simulink model "gm_sampleModel66206_pp_7_1_sub"  (R2023b)
settings: Solver=VariableStepAuto  StartTime=0.0  StopTime=10.0  RelTol=1e-3
libraries: simulink x38, hdlsllib x2, hdlmdlgenlib x2
(part 2 of 2)

== system gm_sampleModel66206_pp_7_1_sub/Subsystem/cfblk35 ==
  emi_178 : Inport  OutDataTypeStr=uint8  PortDimensions=1  SampleTime=1
  Action Port : Inport  Port=2  OutDataTypeStr=boolean  SampleTime=1
  Reshape : Reshape
  cfblk35_out1bypassMux : MultiPortSwitch  DataPortOrder=Zero-based contiguous  Inputs=2  zeroidx=on  OutDataTypeStr=uint8  SampleTime=1  SaturateOnIntegerOverflow=off  InputSameDT=off
  emi_179_bypass : UnitDelay  InitialCondition="fi(0,0,8,0,\"hex\",\"00\")"  SampleTime=1
  emi_179 : Outport  SampleTime=1  InitialOutput=0
  wires:
  Action Port/1 -> cfblk35_out1bypassMux/1
  emi_178/1 -> Reshape/1
  Reshape/1 -> cfblk35_out1bypassMux/3
  cfblk35_out1bypassMux/1 -> emi_179_bypass/1, emi_179/1
  emi_179_bypass/1 -> cfblk35_out1bypassMux/2

== system gm_sampleModel66206_pp_7_1_sub/Subsystem/cfblk36_inst ==
  in1 : Inport  OutDataTypeStr=uint8  SampleTime=1
  in2 : Inport  Port=2  OutDataTypeStr=uint8  SampleTime=1
  mul_cfblk36_dotp_mulcomp : Product  Inputs=**  OutDataTypeStr=uint8  SampleTime=1
  out1 : Outport  OutDataTypeStr=uint8  SampleTime=1
  wires:
  in1/1 -> mul_cfblk36_dotp_mulcomp/1
  in2/1 -> mul_cfblk36_dotp_mulcomp/2
  mul_cfblk36_dotp_mulcomp/1 -> out1/1

== system gm_sampleModel66206_pp_7_1_sub/Subsystem/cfblk40 ==
  u : Inport  OutDataTypeStr=uint8  SampleTime=1
  FixPt Constant : Constant  DisableCoverage=on  OutDataTypeStr=Inherit: Inherit via back propagation  SampleTime=-1
  FixPt Data Type Duplicate : DataTypeDuplicate  DisableCoverage=on  NumInputPorts=3
  FixPt Sum1 : Sum  OutDataTypeStr=Inherit: Inherit via back propagation  InputSameDT=on  LockScale=on
  y : Outport  SampleTime=1
  wires:
  u/1 -> FixPt Sum1/1, FixPt Data Type Duplicate/2
  FixPt Constant/1 -> FixPt Sum1/2, FixPt Data Type Duplicate/3
  FixPt Sum1/1 -> FixPt Data Type Duplicate/1, y/1

== system gm_sampleModel66206_pp_7_1_sub/Subsystem/cfblk42_inst ==
  in1 : Inport  OutDataTypeStr=uint8  SampleTime=1
  in2 : Inport  Port=2  OutDataTypeStr=uint8  SampleTime=1
  mul_cfblk42_dotp_mulcomp : Product  Inputs=**  OutDataTypeStr=uint8  SampleTime=1
  out1 : Outport  OutDataTypeStr=uint8  SampleTime=1
  wires:
  in1/1 -> mul_cfblk42_dotp_mulcomp/1
  in2/1 -> mul_cfblk42_dotp_mulcomp/2
  mul_cfblk42_dotp_mulcomp/1 -> out1/1

== system gm_sampleModel66206_pp_7_1_sub/Subsystem/cfblk44_inst ==
  in1 : Inport  OutDataTypeStr=uint8  SampleTime=1
  in2 : Inport  Port=2  OutDataTypeStr=uint8  SampleTime=1
  mul_cfblk44_dotp_mulcomp : Product  Inputs=**  OutDataTypeStr=uint8  SampleTime=1
  out1 : Outport  OutDataTypeStr=uint8  SampleTime=1
  wires:
  in1/1 -> mul_cfblk44_dotp_mulcomp/1
  in2/1 -> mul_cfblk44_dotp_mulcomp/2
  mul_cfblk44_dotp_mulcomp/1 -> out1/1

== system gm_sampleModel66206_pp_7_1_sub/Subsystem/cfblk47 ==
  emi_186 : Inport  OutDataTypeStr=uint8  PortDimensions=1  SampleTime=1
  Action Port : Inport  Port=2  OutDataTypeStr=boolean  SampleTime=1
  cfblk47 : Sum  Inputs=+
  cfblk47_out1bypassMux : MultiPortSwitch  DataPortOrder=Zero-based contiguous  Inputs=2  zeroidx=on  OutDataTypeStr=uint8  SampleTime=1  SaturateOnIntegerOverflow=off  InputSameDT=off
  emi_187_bypass : UnitDelay  InitialCondition="fi(0,0,8,0,\"hex\",\"00\")"  SampleTime=1
  emi_187 : Outport  SampleTime=1  InitialOutput=0
  wires:
  Action Port/1 -> cfblk47_out1bypassMux/1
  emi_186/1 -> cfblk47/1
  cfblk47/1 -> cfblk47_out1bypassMux/3
  cfblk47_out1bypassMux/1 -> emi_187_bypass/1, emi_187/1
  emi_187_bypass/1 -> cfblk47_out1bypassMux/2

== system gm_sampleModel66206_pp_7_1_sub/Subsystem/cfblk5 ==
  emi_202 : Inport  OutDataTypeStr=fixdt(0, 16, 7)  PortDimensions=1  SampleTime=1
  Action Port : Inport  Port=2  OutDataTypeStr=boolean  SampleTime=1
  cfblk5 : Subsystem  mask(Detect Fall Nonpositive){vinit=double(0), InputProcessing=Elements as channels (sample based), OutDataTypeStr=uint8}
      mask prompts: vinit "Simulink:masks:InitialCondition_MP"; InputProcessing "Simulink:masks:InputProcessing_MP"; OutDataTypeStr "Simulink:masks:OutputDataType_MP"
      mask help: Simulink:masks:DetectFallNonpositive_MD
      mask TypeOptions InputProcessing: Simulink:masks:ColumnsAsChannelsFrameBased | Simulink:masks:ElementsAsChannelsSampleBased
      mask TypeOptions OutDataTypeStr: Simulink:masks:uint8 | Simulink:masks:boolean
      mask Display: fprintf('U <= 0\n&  NOT\nU/z <= 0')
  cfblk5_out1bypassMux : MultiPortSwitch  DataPortOrder=Zero-based contiguous  Inputs=2  zeroidx=on  OutDataTypeStr=uint8  SampleTime=1  SaturateOnIntegerOverflow=off  InputSameDT=off
  emi_203_bypass : UnitDelay  InitialCondition="fi(0,0,8,0,\"hex\",\"00\")"  SampleTime=1
  emi_203 : Outport  SampleTime=1  InitialOutput=0
  wires:
  Action Port/1 -> cfblk5_out1bypassMux/1, cfblk5/2(Action Port_out2)
  emi_202/1 -> cfblk5/1(U)
  cfblk5/1(Y) -> cfblk5_out1bypassMux/3
  cfblk5_out1bypassMux/1 -> emi_203_bypass/1, emi_203/1
  emi_203_bypass/1 -> cfblk5_out1bypassMux/2

== system gm_sampleModel66206_pp_7_1_sub/Subsystem/cfblk50 ==
  emi_210 : Inport  OutDataTypeStr=uint8  PortDimensions=1  SampleTime=1
  Action Port : Inport  Port=2  OutDataTypeStr=boolean  SampleTime=1
  cfblk50 : Gain  Gain="fi(0,0,8,7,\"hex\",\"80\")"  ParamDataTypeStr=fixdt(0, 8, 7)  OutDataTypeStr=fixdt(0, 16, 7)  SampleTime=1
  cfblk50_out1bypassMux : MultiPortSwitch  DataPortOrder=Zero-based contiguous  Inputs=2  zeroidx=on  OutDataTypeStr=fixdt(0, 16, 7)  SampleTime=1  SaturateOnIntegerOverflow=off  InputSameDT=off
  emi_211_bypass : UnitDelay  InitialCondition="fi(0,0,16,7,\"hex\",\"0000\")"  SampleTime=1
  emi_211 : Outport  SampleTime=1  InitialOutput=0
  wires:
  Action Port/1 -> cfblk50_out1bypassMux/1
  emi_210/1 -> cfblk50/1
  cfblk50/1 -> cfblk50_out1bypassMux/3
  cfblk50_out1bypassMux/1 -> emi_211_bypass/1, emi_211/1
  emi_211_bypass/1 -> cfblk50_out1bypassMux/2

== system gm_sampleModel66206_pp_7_1_sub/Subsystem/cfblk51 ==
  emi_218 : Inport  OutDataTypeStr=uint8  PortDimensions=1  SampleTime=1
  Action Port : Inport  Port=2  OutDataTypeStr=boolean  SampleTime=1
  cfblk51 : Subsystem  mask(Real World Value Increment){}
      mask help: Simulink:masks:RealWorldValueIncrement_MD
      mask Display: disp('V++')
  cfblk51_out1bypassMux : MultiPortSwitch  DataPortOrder=Zero-based contiguous  Inputs=2  zeroidx=on  OutDataTypeStr=uint8  SampleTime=1  SaturateOnIntegerOverflow=off  InputSameDT=off
  emi_219_bypass : UnitDelay  InitialCondition="fi(0,0,8,0,\"hex\",\"00\")"  SampleTime=1
  emi_219 : Outport  SampleTime=1  InitialOutput=0
  wires:
  Action Port/1 -> cfblk51_out1bypassMux/1
  emi_218/1 -> cfblk51/1(u)
  cfblk51/1(y) -> cfblk51_out1bypassMux/3
  cfblk51_out1bypassMux/1 -> emi_219_bypass/1, emi_219/1
  emi_219_bypass/1 -> cfblk51_out1bypassMux/2

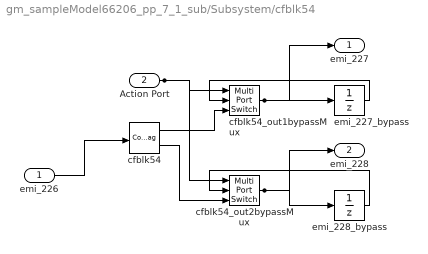
== system gm_sampleModel66206_pp_7_1_sub/Subsystem/cfblk54 ==
  emi_226 : Inport  OutDataTypeStr=uint8  PortDimensions=1  SampleTime=1
  Action Port : Inport  Port=2  OutDataTypeStr=boolean  SampleTime=1
  cfblk54 : ComplexToRealImag  SampleTime=1
  cfblk54_out1bypassMux : MultiPortSwitch  DataPortOrder=Zero-based contiguous  Inputs=2  zeroidx=on  OutDataTypeStr=uint8  SampleTime=1  SaturateOnIntegerOverflow=off  InputSameDT=off
  cfblk54_out2bypassMux : MultiPortSwitch  DataPortOrder=Zero-based contiguous  Inputs=2  zeroidx=on  OutDataTypeStr=uint8  SampleTime=1  SaturateOnIntegerOverflow=off  InputSameDT=off
  emi_227_bypass : UnitDelay  InitialCondition="fi(0,0,8,0,\"hex\",\"00\")"  SampleTime=1
  emi_228_bypass : UnitDelay  InitialCondition="fi(0,0,8,0,\"hex\",\"00\")"  SampleTime=1
  emi_227 : Outport  SampleTime=1  InitialOutput=0
  emi_228 : Outport  Port=2  SampleTime=1  InitialOutput=0
  wires:
  Action Port/1 -> cfblk54_out2bypassMux/1, cfblk54_out1bypassMux/1
  emi_226/1 -> cfblk54/1
  cfblk54/1 -> cfblk54_out1bypassMux/3
  cfblk54/2 -> cfblk54_out2bypassMux/3
  cfblk54_out1bypassMux/1 -> emi_227_bypass/1, emi_227/1
  emi_227_bypass/1 -> cfblk54_out1bypassMux/2
  cfblk54_out2bypassMux/1 -> emi_228_bypass/1, emi_228/1
  emi_228_bypass/1 -> cfblk54_out2bypassMux/2

== system gm_sampleModel66206_pp_7_1_sub/Subsystem/cfblk55 ==
  emi_235 : Inport  OutDataTypeStr=uint8  PortDimensions=1  SampleTime=1
  Action Port : Inport  Port=2  OutDataTypeStr=boolean  SampleTime=1
  cfblk55 : Abs  SampleTime=1  OutDataTypeStr=uint8  SaturateOnIntegerOverflow=off
  cfblk55_out1bypassMux : MultiPortSwitch  DataPortOrder=Zero-based contiguous  Inputs=2  zeroidx=on  OutDataTypeStr=uint8  SampleTime=1  SaturateOnIntegerOverflow=off  InputSameDT=off
  emi_236_bypass : UnitDelay  InitialCondition="fi(0,0,8,0,\"hex\",\"00\")"  SampleTime=1
  emi_236 : Outport  SampleTime=1  InitialOutput=0
  wires:
  Action Port/1 -> cfblk55_out1bypassMux/1
  emi_235/1 -> cfblk55/1
  cfblk55/1 -> cfblk55_out1bypassMux/3
  cfblk55_out1bypassMux/1 -> emi_236_bypass/1, emi_236/1
  emi_236_bypass/1 -> cfblk55_out1bypassMux/2

== system gm_sampleModel66206_pp_7_1_sub/Subsystem/cfblk59 ==
  u : Inport  OutDataTypeStr=uint8  SampleTime=1
  FixPt Constant : Constant  DisableCoverage=on  OutDataTypeStr=Inherit: Inherit via back propagation  SampleTime=-1
  FixPt Data Type Duplicate : DataTypeDuplicate  DisableCoverage=on  NumInputPorts=3
  FixPt Sum1 : Sum  OutDataTypeStr=Inherit: Inherit via back propagation  InputSameDT=on  LockScale=on
  y : Outport  SampleTime=1
  wires:
  u/1 -> FixPt Sum1/1, FixPt Data Type Duplicate/2
  FixPt Constant/1 -> FixPt Sum1/2, FixPt Data Type Duplicate/3
  FixPt Sum1/1 -> FixPt Data Type Duplicate/1, y/1

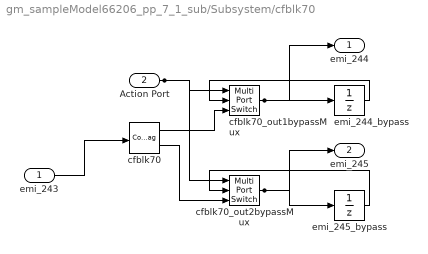
== system gm_sampleModel66206_pp_7_1_sub/Subsystem/cfblk70 ==
  emi_243 : Inport  OutDataTypeStr=uint8  PortDimensions=1  SampleTime=1
  Action Port : Inport  Port=2  OutDataTypeStr=boolean  SampleTime=1
  cfblk70 : ComplexToRealImag  SampleTime=1
  cfblk70_out1bypassMux : MultiPortSwitch  DataPortOrder=Zero-based contiguous  Inputs=2  zeroidx=on  OutDataTypeStr=uint8  SampleTime=1  SaturateOnIntegerOverflow=off  InputSameDT=off
  cfblk70_out2bypassMux : MultiPortSwitch  DataPortOrder=Zero-based contiguous  Inputs=2  zeroidx=on  OutDataTypeStr=uint8  SampleTime=1  SaturateOnIntegerOverflow=off  InputSameDT=off
  emi_244_bypass : UnitDelay  InitialCondition="fi(0,0,8,0,\"hex\",\"00\")"  SampleTime=1
  emi_245_bypass : UnitDelay  InitialCondition="fi(0,0,8,0,\"hex\",\"00\")"  SampleTime=1
  emi_244 : Outport  SampleTime=1  InitialOutput=0
  emi_245 : Outport  Port=2  SampleTime=1  InitialOutput=0
  wires:
  Action Port/1 -> cfblk70_out2bypassMux/1, cfblk70_out1bypassMux/1
  emi_243/1 -> cfblk70/1
  cfblk70/1 -> cfblk70_out1bypassMux/3
  cfblk70/2 -> cfblk70_out2bypassMux/3
  cfblk70_out1bypassMux/1 -> emi_244_bypass/1, emi_244/1
  emi_244_bypass/1 -> cfblk70_out1bypassMux/2
  cfblk70_out2bypassMux/1 -> emi_245_bypass/1, emi_245/1
  emi_245_bypass/1 -> cfblk70_out2bypassMux/2

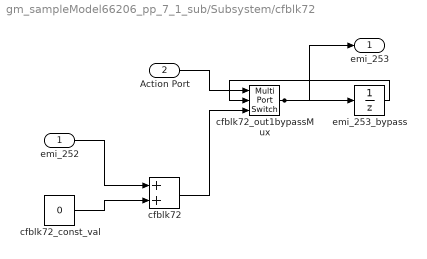
== system gm_sampleModel66206_pp_7_1_sub/Subsystem/cfblk72 ==
  emi_252 : Inport  OutDataTypeStr=uint8  PortDimensions=1  SampleTime=1
  Action Port : Inport  Port=2  OutDataTypeStr=boolean  SampleTime=1
  cfblk72 : Sum  OutDataTypeStr=uint8  AccumDataTypeStr=uint8  RndMeth=Nearest  SampleTime=1
  cfblk72_const_val : Constant  Value=0  VectorParams1D=off  OutDataTypeStr=uint8  SampleTime=1
  cfblk72_out1bypassMux : MultiPortSwitch  DataPortOrder=Zero-based contiguous  Inputs=2  zeroidx=on  OutDataTypeStr=uint8  SampleTime=1  SaturateOnIntegerOverflow=off  InputSameDT=off
  emi_253_bypass : UnitDelay  InitialCondition="fi(0,0,8,0,\"hex\",\"00\")"  SampleTime=1
  emi_253 : Outport  SampleTime=1  InitialOutput=0
  wires:
  Action Port/1 -> cfblk72_out1bypassMux/1
  emi_252/1 -> cfblk72/1
  cfblk72/1 -> cfblk72_out1bypassMux/3
  cfblk72_out1bypassMux/1 -> emi_253_bypass/1, emi_253/1
  emi_253_bypass/1 -> cfblk72_out1bypassMux/2
  cfblk72_const_val/1 -> cfblk72/2

== system gm_sampleModel66206_pp_7_1_sub/Subsystem/cfblk74 ==
  emi_260 : Inport  OutDataTypeStr=uint8  PortDimensions=1  SampleTime=1
  Action Port : Inport  Port=2  OutDataTypeStr=boolean  SampleTime=1
  cfblk74 : Sum  Inputs=+
  cfblk74_out1bypassMux : MultiPortSwitch  DataPortOrder=Zero-based contiguous  Inputs=2  zeroidx=on  OutDataTypeStr=uint8  SampleTime=1  SaturateOnIntegerOverflow=off  InputSameDT=off
  emi_261_bypass : UnitDelay  InitialCondition="fi(0,0,8,0,\"hex\",\"00\")"  SampleTime=1
  emi_261 : Outport  SampleTime=1  InitialOutput=0
  wires:
  Action Port/1 -> cfblk74_out1bypassMux/1
  emi_260/1 -> cfblk74/1
  cfblk74/1 -> cfblk74_out1bypassMux/3
  cfblk74_out1bypassMux/1 -> emi_261_bypass/1, emi_261/1
  emi_261_bypass/1 -> cfblk74_out1bypassMux/2

== system gm_sampleModel66206_pp_7_1_sub/Subsystem/cfblk80 ==
  u : Inport  OutDataTypeStr=uint8  SampleTime=1
  FixPt Constant : Constant  DisableCoverage=on  OutDataTypeStr=Inherit: Inherit via back propagation  SampleTime=-1
  FixPt Data Type Duplicate : DataTypeDuplicate  DisableCoverage=on  NumInputPorts=3
  FixPt Sum1 : Sum  OutDataTypeStr=Inherit: Inherit via back propagation  InputSameDT=on  LockScale=on
  y : Outport  SampleTime=1
  wires:
  u/1 -> FixPt Sum1/1, FixPt Data Type Duplicate/2
  FixPt Constant/1 -> FixPt Sum1/2, FixPt Data Type Duplicate/3
  FixPt Sum1/1 -> FixPt Data Type Duplicate/1, y/1

== system gm_sampleModel66206_pp_7_1_sub/Subsystem/cfblk84 ==
  emi_82 : Inport  OutDataTypeStr=uint8  PortDimensions=1  SampleTime=1
  Action Port : Inport  Port=2  OutDataTypeStr=boolean  SampleTime=1
  cfblk84 : Abs  SampleTime=1  OutDataTypeStr=uint8  SaturateOnIntegerOverflow=off
  cfblk84_out1bypassMux : MultiPortSwitch  DataPortOrder=Zero-based contiguous  Inputs=2  zeroidx=on  OutDataTypeStr=uint8  SampleTime=1  SaturateOnIntegerOverflow=off  InputSameDT=off
  emi_83_bypass : UnitDelay  InitialCondition="fi(0,0,8,0,\"hex\",\"00\")"  SampleTime=1
  emi_83 : Outport  SampleTime=1  InitialOutput=0
  wires:
  Action Port/1 -> cfblk84_out1bypassMux/1
  emi_82/1 -> cfblk84/1
  cfblk84/1 -> cfblk84_out1bypassMux/3
  cfblk84_out1bypassMux/1 -> emi_83_bypass/1, emi_83/1
  emi_83_bypass/1 -> cfblk84_out1bypassMux/2

== system gm_sampleModel66206_pp_7_1_sub/Subsystem/cfblk92 ==
  emi_276 : Inport  OutDataTypeStr=uint8  PortDimensions=1  SampleTime=1
  Action Port : Inport  Port=2  OutDataTypeStr=boolean  SampleTime=1
  cfblk92 : MinMax
  cfblk92_out1bypassMux : MultiPortSwitch  DataPortOrder=Zero-based contiguous  Inputs=2  zeroidx=on  OutDataTypeStr=uint8  SampleTime=1  SaturateOnIntegerOverflow=off  InputSameDT=off
  emi_277_bypass : UnitDelay  InitialCondition="fi(0,0,8,0,\"hex\",\"00\")"  SampleTime=1
  emi_277 : Outport  SampleTime=1  InitialOutput=0
  wires:
  Action Port/1 -> cfblk92_out1bypassMux/1
  emi_276/1 -> cfblk92/1
  cfblk92/1 -> cfblk92_out1bypassMux/3
  cfblk92_out1bypassMux/1 -> emi_277_bypass/1, emi_277/1
  emi_277_bypass/1 -> cfblk92_out1bypassMux/2

== system gm_sampleModel66206_pp_7_1_sub/Subsystem/cfblk94_inst ==
  in1 : Inport  OutDataTypeStr=uint8  SampleTime=1
  in2 : Inport  Port=2  OutDataTypeStr=uint8  SampleTime=1
  mul_cfblk94_dotp_mulcomp : Product  Inputs=**  OutDataTypeStr=uint8  SampleTime=1
  out1 : Outport  OutDataTypeStr=uint8  SampleTime=1
  wires:
  in1/1 -> mul_cfblk94_dotp_mulcomp/1
  in2/1 -> mul_cfblk94_dotp_mulcomp/2
  mul_cfblk94_dotp_mulcomp/1 -> out1/1

== system gm_sampleModel66206_pp_7_1_sub/Subsystem/cfblk96 ==
  emi_284 : Inport  OutDataTypeStr=uint8  PortDimensions=1  SampleTime=1
  Action Port : Inport  Port=2  OutDataTypeStr=boolean  SampleTime=1
  cfblk96 : Sum  Inputs=+
  cfblk96_out1bypassMux : MultiPortSwitch  DataPortOrder=Zero-based contiguous  Inputs=2  zeroidx=on  OutDataTypeStr=uint8  SampleTime=1  SaturateOnIntegerOverflow=off  InputSameDT=off
  emi_285_bypass : UnitDelay  InitialCondition="fi(0,0,8,0,\"hex\",\"00\")"  SampleTime=1
  emi_285 : Outport  SampleTime=1  InitialOutput=0
  wires:
  Action Port/1 -> cfblk96_out1bypassMux/1
  emi_284/1 -> cfblk96/1
  cfblk96/1 -> cfblk96_out1bypassMux/3
  cfblk96_out1bypassMux/1 -> emi_285_bypass/1, emi_285/1
  emi_285_bypass/1 -> cfblk96_out1bypassMux/2

== system gm_sampleModel66206_pp_7_1_sub/Subsystem/cfblk1/Nonpositive ==
  u : Inport  OutDataTypeStr=uint8  SampleTime=1
  Compare : RelationalOperator  Operator=<=  OutDataTypeStr=boolean  ZeroCross=off
  Constant : Constant  DisableCoverage=on  Value=0  OutDataTypeStr=Inherit: Inherit via back propagation  SampleTime=-1  PreserveConstantTs=on
  y : Outport  SampleTime=1
  wires:
  u/1 -> Compare/1
  Compare/1 -> y/1
  Constant/1 -> Compare/2

== system gm_sampleModel66206_pp_7_1_sub/Subsystem/cfblk10/Positive ==
  u : Inport  OutDataTypeStr=uint8  SampleTime=1
  Compare : RelationalOperator  Operator=>  OutDataTypeStr=boolean  ZeroCross=off
  Constant : Constant  DisableCoverage=on  Value=0  OutDataTypeStr=Inherit: Inherit via back propagation  SampleTime=-1  PreserveConstantTs=on
  y : Outport  SampleTime=1
  wires:
  u/1 -> Compare/1
  Compare/1 -> y/1
  Constant/1 -> Compare/2

== system gm_sampleModel66206_pp_7_1_sub/Subsystem/cfblk11/Nonpositive ==
  u : Inport  OutDataTypeStr=uint8  SampleTime=1
  Compare : RelationalOperator  Operator=<=  OutDataTypeStr=boolean  ZeroCross=off
  Constant : Constant  DisableCoverage=on  Value=0  OutDataTypeStr=Inherit: Inherit via back propagation  SampleTime=-1  PreserveConstantTs=on
  y : Outport  SampleTime=1
  wires:
  u/1 -> Compare/1
  Compare/1 -> y/1
  Constant/1 -> Compare/2

== system gm_sampleModel66206_pp_7_1_sub/Subsystem/cfblk117/cfblk117 ==
  u : Inport  OutDataTypeStr=uint8  SampleTime=1
  FixPt Constant : Constant  DisableCoverage=on  OutDataTypeStr=Inherit: Inherit via back propagation  SampleTime=-1
  FixPt Data Type Duplicate : DataTypeDuplicate  DisableCoverage=on  NumInputPorts=3
  FixPt Sum1 : Sum  OutDataTypeStr=Inherit: Inherit via back propagation  InputSameDT=on  LockScale=on
  y : Outport  SampleTime=1  InitialOutput=0
  wires:
  u/1 -> FixPt Sum1/1, FixPt Data Type Duplicate/2
  FixPt Constant/1 -> FixPt Sum1/2, FixPt Data Type Duplicate/3
  FixPt Sum1/1 -> FixPt Data Type Duplicate/1, y/1

== system gm_sampleModel66206_pp_7_1_sub/Subsystem/cfblk13/cfblk13 ==
  note: U(k)
  note: Edge
  U : Inport  OutDataTypeStr=uint8  SampleTime=1
  Action Port_out2 : Inport  Port=2  OutDataTypeStr=boolean  SampleTime=1
  Delay Input1 : Subsystem
      settings: MinAlgLoopOccurrences=on
  FixPt Relational Operator : RelationalOperator  Operator=>  OutDataTypeStr=fixdt(0,8,0)  SampleTime=1  InputSameDT=off
  Nonnegative : Subsystem  mask(Compare To Zero){relop=>=, OutDataTypeStr=boolean, ZeroCross=off}
      mask prompts: relop "Simulink:masks:Operator_MP"; OutDataTypeStr "Simulink:masks:OutputDataType_MP"; ZeroCross "Simulink:masks:EnableZerocrossingDetection_MP"
      mask help: Simulink:masks:CompareToZero_MD
      mask TypeOptions relop: == | ~= | < | <= | >= | >
      mask TypeOptions OutDataTypeStr: Simulink:masks:uint8 | Simulink:masks:boolean
      mask Callback ZeroCross: sl('zeroCrossEnable', gcbh);
      mask Display: disp([relop,' 0'])
  Y : Outport  SampleTime=1  InitialOutput=0
  wires:
  U/1 -> Nonnegative/1(u)
  Delay Input1/1(out0) -> FixPt Relational Operator/2
  FixPt Relational Operator/1 -> Y/1
  Nonnegative/1(y) -> FixPt Relational Operator/1, Delay Input1/1(in0)
  Action Port_out2/1 -> Delay Input1/Enable

== system gm_sampleModel66206_pp_7_1_sub/Subsystem/cfblk130/cfblk130 ==
  u : Inport  OutDataTypeStr=uint8  SampleTime=1
  FixPt Constant : Constant  DisableCoverage=on  OutDataTypeStr=Inherit: Inherit via back propagation  SampleTime=-1
  FixPt Data Type Duplicate : DataTypeDuplicate  DisableCoverage=on  NumInputPorts=3
  FixPt Sum1 : Sum  OutDataTypeStr=Inherit: Inherit via back propagation  InputSameDT=on  LockScale=on
  y : Outport  SampleTime=1  InitialOutput=0
  wires:
  u/1 -> FixPt Sum1/1, FixPt Data Type Duplicate/2
  FixPt Constant/1 -> FixPt Sum1/2, FixPt Data Type Duplicate/3
  FixPt Sum1/1 -> FixPt Data Type Duplicate/1, y/1

== system gm_sampleModel66206_pp_7_1_sub/Subsystem/cfblk168/cfblk168 ==
  in0 : Inport  OutDataTypeStr=uint8  SampleTime=1
  Action Port_out2 : EnablePort  OutDataTypeStr=boolean
  cfblk168 : Delay  DelayLength=double(2)  InitialCondition=0
  out0 : Outport  OutDataTypeStr=uint8  SampleTime=1  InitialOutput=0
  wires:
  cfblk168/1 -> out0/1
  in0/1 -> cfblk168/1

== system gm_sampleModel66206_pp_7_1_sub/Subsystem/cfblk2/cfblk2 ==
  note: Edge
  note: U(k)
  U : Inport  OutDataTypeStr=uint8  SampleTime=1
  Action Port_out2 : Inport  Port=2  OutDataTypeStr=boolean  SampleTime=1
  Delay Input1 : Subsystem
      settings: MinAlgLoopOccurrences=on
  FixPt Relational Operator : RelationalOperator  Operator=>  OutDataTypeStr=fixdt(0,8,0)  SampleTime=1  InputSameDT=off
  Y : Outport  SampleTime=1  InitialOutput=0
  wires:
  U/1 -> FixPt Relational Operator/1, Delay Input1/1(in0)
  Delay Input1/1(out0) -> FixPt Relational Operator/2
  FixPt Relational Operator/1 -> Y/1
  Action Port_out2/1 -> Delay Input1/Enable

== system gm_sampleModel66206_pp_7_1_sub/Subsystem/cfblk21/cfblk21 ==
  u : Inport  OutDataTypeStr=uint8  SampleTime=1
  FixPt Constant : Constant  DisableCoverage=on  OutDataTypeStr=Inherit: Inherit via back propagation  SampleTime=-1
  FixPt Data Type Duplicate : DataTypeDuplicate  DisableCoverage=on  NumInputPorts=3
  FixPt Sum1 : Sum  OutDataTypeStr=Inherit: Inherit via back propagation  InputSameDT=on  LockScale=on
  y : Outport  SampleTime=1  InitialOutput=0
  wires:
  u/1 -> FixPt Sum1/1, FixPt Data Type Duplicate/2
  FixPt Constant/1 -> FixPt Sum1/2, FixPt Data Type Duplicate/3
  FixPt Sum1/1 -> FixPt Data Type Duplicate/1, y/1

== system gm_sampleModel66206_pp_7_1_sub/Subsystem/cfblk28/cfblk28 ==
  u : Inport  OutDataTypeStr=uint8  SampleTime=1
  FixPt Constant : Constant  DisableCoverage=on  OutDataTypeStr=Inherit: Inherit via back propagation  SampleTime=-1
  FixPt Data Type Duplicate : DataTypeDuplicate  DisableCoverage=on  NumInputPorts=3
  FixPt Sum1 : Sum  OutDataTypeStr=Inherit: Inherit via back propagation  InputSameDT=on  LockScale=on
  y : Outport  SampleTime=1  InitialOutput=0
  wires:
  u/1 -> FixPt Sum1/1, FixPt Data Type Duplicate/2
  FixPt Constant/1 -> FixPt Sum1/2, FixPt Data Type Duplicate/3
  FixPt Sum1/1 -> FixPt Data Type Duplicate/1, y/1

== system gm_sampleModel66206_pp_7_1_sub/Subsystem/cfblk5/cfblk5 ==
  note: U(k)
  note: Edge
  U : Inport  OutDataTypeStr=fixdt(0, 16, 7)  SampleTime=1
  Action Port_out2 : Inport  Port=2  OutDataTypeStr=boolean  SampleTime=1
  Delay Input1 : Subsystem
      settings: MinAlgLoopOccurrences=on
  FixPt Relational Operator : RelationalOperator  Operator=>  OutDataTypeStr=fixdt(0,8,0)  SampleTime=1  InputSameDT=off
  Nonpositive : Subsystem  mask(Compare To Zero){relop=<=, OutDataTypeStr=boolean, ZeroCross=off}
      mask prompts: relop "Simulink:masks:Operator_MP"; OutDataTypeStr "Simulink:masks:OutputDataType_MP"; ZeroCross "Simulink:masks:EnableZerocrossingDetection_MP"
      mask help: Simulink:masks:CompareToZero_MD
      mask TypeOptions relop: == | ~= | < | <= | >= | >
      mask TypeOptions OutDataTypeStr: Simulink:masks:uint8 | Simulink:masks:boolean
      mask Callback ZeroCross: sl('zeroCrossEnable', gcbh);
      mask Display: disp([relop,' 0'])
  Y : Outport  SampleTime=1  InitialOutput=0
  wires:
  U/1 -> Nonpositive/1(u)
  Delay Input1/1(out0) -> FixPt Relational Operator/2
  FixPt Relational Operator/1 -> Y/1
  Nonpositive/1(y) -> FixPt Relational Operator/1, Delay Input1/1(in0)
  Action Port_out2/1 -> Delay Input1/Enable

== system gm_sampleModel66206_pp_7_1_sub/Subsystem/cfblk51/cfblk51 ==
  u : Inport  OutDataTypeStr=uint8  SampleTime=1
  FixPt Constant : Constant  DisableCoverage=on  OutDataTypeStr=Inherit: Inherit via back propagation  SampleTime=-1
  FixPt Data Type Duplicate : DataTypeDuplicate  DisableCoverage=on  NumInputPorts=3
  FixPt Sum1 : Sum  OutDataTypeStr=Inherit: Inherit via back propagation  InputSameDT=on  LockScale=on
  y : Outport  SampleTime=1  InitialOutput=0
  wires:
  u/1 -> FixPt Sum1/1, FixPt Data Type Duplicate/2
  FixPt Constant/1 -> FixPt Sum1/2, FixPt Data Type Duplicate/3
  FixPt Sum1/1 -> FixPt Data Type Duplicate/1, y/1

== system gm_sampleModel66206_pp_7_1_sub/Subsystem/cfblk13/cfblk13/Delay Input1 ==
  in0 : Inport  OutDataTypeStr=boolean  SampleTime=1
  Action Port_out2 : EnablePort  OutDataTypeStr=boolean
  Delay Input1 : UnitDelay  SampleTime=1
  out0 : Outport  OutDataTypeStr=boolean  SampleTime=1  InitialOutput=0
  wires:
  Delay Input1/1 -> out0/1
  in0/1 -> Delay Input1/1

== system gm_sampleModel66206_pp_7_1_sub/Subsystem/cfblk13/cfblk13/Nonnegative ==
  u : Inport  OutDataTypeStr=uint8  SampleTime=1
  Compare : RelationalOperator  OutDataTypeStr=boolean  SampleTime=1
  Constant : Constant  Value=0  OutDataTypeStr=uint8  SampleTime=1
  y : Outport  SampleTime=1  InitialOutput=0
  wires:
  u/1 -> Compare/1
  Compare/1 -> y/1
  Constant/1 -> Compare/2

== system gm_sampleModel66206_pp_7_1_sub/Subsystem/cfblk2/cfblk2/Delay Input1 ==
  in0 : Inport  OutDataTypeStr=uint8  SampleTime=1
  Action Port_out2 : EnablePort  OutDataTypeStr=boolean
  Delay Input1 : Delay  DelayLength=double(1)  InitialCondition=0
  out0 : Outport  OutDataTypeStr=uint8  SampleTime=1  InitialOutput=0
  wires:
  Delay Input1/1 -> out0/1
  in0/1 -> Delay Input1/1

== system gm_sampleModel66206_pp_7_1_sub/Subsystem/cfblk5/cfblk5/Delay Input1 ==
  in0 : Inport  OutDataTypeStr=boolean  SampleTime=1
  Action Port_out2 : EnablePort  OutDataTypeStr=boolean
  Delay Input1 : UnitDelay  SampleTime=1
  out0 : Outport  OutDataTypeStr=boolean  SampleTime=1  InitialOutput=0
  wires:
  Delay Input1/1 -> out0/1
  in0/1 -> Delay Input1/1

== system gm_sampleModel66206_pp_7_1_sub/Subsystem/cfblk5/cfblk5/Nonpositive ==
  u : Inport  OutDataTypeStr=fixdt(0, 16, 7)  SampleTime=1
  Compare : RelationalOperator  Operator=<=  OutDataTypeStr=boolean  SampleTime=1
  Constant : Constant  Value=0  OutDataTypeStr=fixdt(0, 16, 7)  SampleTime=1
  y : Outport  SampleTime=1  InitialOutput=0
  wires:
  u/1 -> Compare/1
  Compare/1 -> y/1
  Constant/1 -> Compare/2
